simulink model "NDS_SKF"  (R2022b)
settings: Solver=ode4  StartTime=0.0  StopTime=10  RelTol=1e-3
values from neighbouring files (symbols this model uses):
  A = [(-2 * DCR * wn) -(wn^2); 1 0]    [NDS_SKFmat.m]
  B = [wn^2; 0]    [NDS_SKFmat.m]
  F_k1 = sys_d.A    [NDS_SKFmat.m]
  G_k1 = sys_d.B    [NDS_SKFmat.m]
  H_k1 = sys_d.C    [NDS_SKFmat.m]
  L_k1 = G_k1    [NDS_SKFmat.m]
  M_k1 = 1    [NDS_SKFmat.m]
  Pk0 = eye(size(xhat0, 1))    [NDS_SKFmat.m]
  Q = 0.1    [NDS_SKFmat.m]
  R = 0.1    [NDS_SKFmat.m]
  x0 = 0.5    [NDS_SKFmat.m]
  xdot0 = -0.01    [NDS_SKFmat.m]
  xhat0 = [0; 0]    [NDS_SKFmat.m]
settings Model: Creator=nathaliadesouza  LastModifiedBy=nathaliadesouza

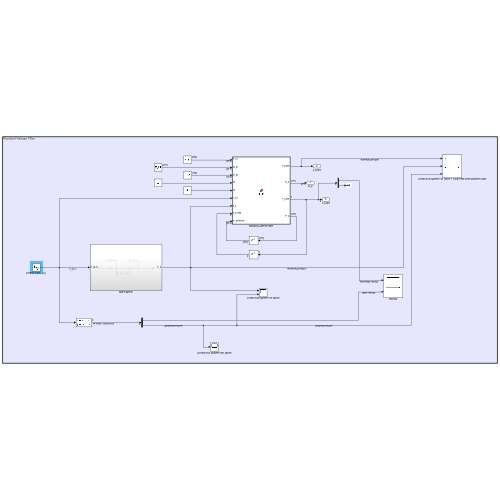
[thumbnail: Simulink's stored preview of the top-level diagram]
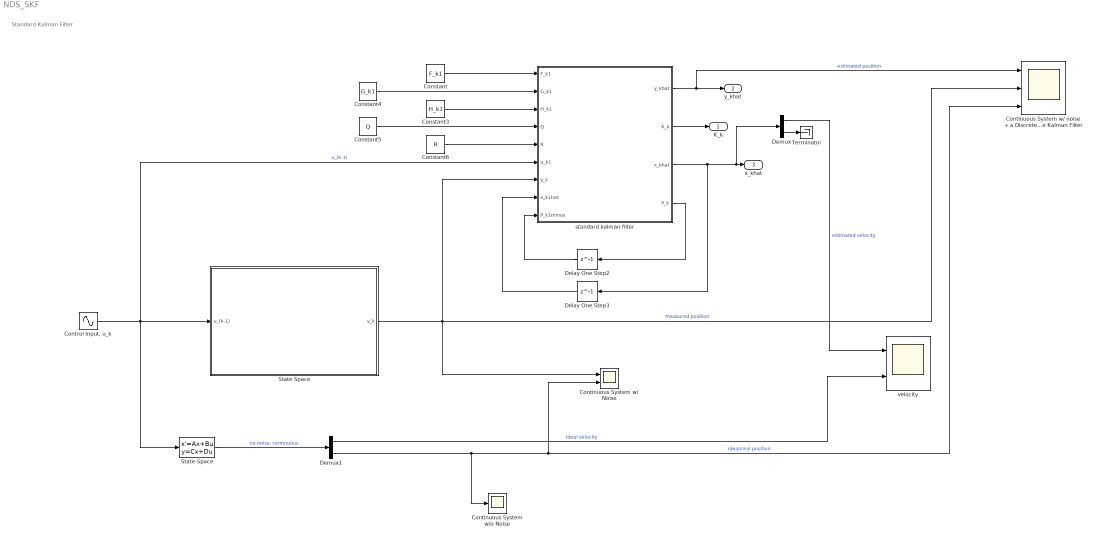
== system NDS_SKF ==
  note: Standard Kalman Filter
  Constant : Constant  Value=F_k1  VectorParams1D=off
  Constant3 : Constant  Value=H_k1  VectorParams1D=off
  Constant4 : Constant  Value=G_k1  VectorParams1D=off
  Constant5 : Constant  Value=Q
  Constant6 : Constant  Value=R
  Continuous System w/ Noise : Scope  NumInputPorts=2
  Continuous System w/ noise + a Discrete Time Kalman Filter : Scope  NumInputPorts=3
  Continuous System w/o Noise : Scope
  "Control Input, u_k " : Sin  SampleTime=0.1
  Delay One Step2 : Delay  DelayLength=1  InitialCondition=Pk0  SampleTime=0.1
  Delay One Step3 : Delay  DelayLength=1  InitialCondition=xhat0  SampleTime=0.1
  Demux : Demux  Outputs=2
  Demux1 : Demux  Outputs=2
  State Space : Subsystem
  State-Space : StateSpace  A=A  B=B  C=eye(2)  D=[0; 0]  InitialCondition=[x0 xdot0]
  Terminator : Terminator
  standard kalman filter : MATLAB Function  TreatAsAtomicUnit=on
  velocity : Scope  NumInputPorts=2
  K_k : Outport
  y_khat : Outport  Port=2
  x_khat : Outport  Port=3
  wires:
  "Control Input, u_k "/1 -> standard kalman filter/6(u_k1), State Space/1(u_(k-1)), State-Space/1  "u_(k-1)"
  Constant4/1 -> standard kalman filter/2(G_k1)
  Constant5/1 -> standard kalman filter/4(Q)
  Constant/1 -> standard kalman filter/1(F_k1)
  Constant6/1 -> standard kalman filter/5(R)
  Constant3/1 -> standard kalman filter/3(H_k1)
  standard kalman filter/3(x_khat) -> Delay One Step3/1, Demux/1, x_khat/1
  Delay One Step2/1 -> standard kalman filter/9(P_k1minus)
  Delay One Step3/1 -> standard kalman filter/8(x_k1hat)
  standard kalman filter/4(P_k) -> Delay One Step2/1
  standard kalman filter/1(y_khat) -> Continuous System w/ noise + a Discrete Time Kalman Filter/1, y_khat/1  "estimated position"
  standard kalman filter/2(K_k) -> K_k/1
  State-Space/1 -> Demux1/1  "no noise, continuous"
  Demux1/2 -> Continuous System w/o Noise/1, Continuous System w/ Noise/2, Continuous System w/ noise + a Discrete Time Kalman Filter/3  "ideal/real position"
  Demux1/1 -> velocity/2  "ideal velocity"
  Demux/1 -> velocity/1  "estimated velocity"
  Demux/2 -> Terminator/1
  State Space/1(y_k) -> standard kalman filter/7(y_k), Continuous System w/ Noise/1, Continuous System w/ noise + a Discrete Time Kalman Filter/2  "measured position"

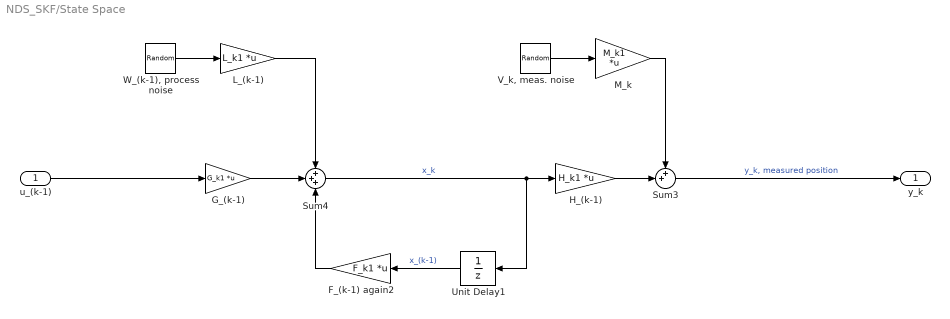
== system NDS_SKF/State Space ==
  u_(k-1) : Inport
  F_(k-1) again2 : Gain  Gain=F_k1  Multiplication=Matrix(K*u)
  G_(k-1) : Gain  Gain=G_k1  Multiplication=Matrix(K*u)
  H_(k-1) : Gain  Gain=H_k1  Multiplication=Matrix(K*u)
  L_(k-1) : Gain  Gain=L_k1  Multiplication=Matrix(K*u)  SampleTime=0.1
  M_k : Gain  Gain=M_k1  Multiplication=Matrix(K*u)  SampleTime=0.1
  Sum3 : Sum  Inputs=++|
  Sum4 : Sum  Inputs=+++
  Unit Delay1 : UnitDelay  InitialCondition=[0.5; -0.01]  SampleTime=0.1  HasFrameUpgradeWarning=on
  "V_k, meas. noise" : RandomNumber  Variance=0.01  SampleTime=0.1
  "W_(k-1), process noise" : RandomNumber  Variance=0.01  SampleTime=0.1
  y_k : Outport
  wires:
  u_(k-1)/1 -> G_(k-1)/1
  L_(k-1)/1 -> Sum4/1
  Unit Delay1/1 -> F_(k-1) again2/1  "x_(k-1)"
  "V_k, meas. noise"/1 -> M_k/1
  Sum4/1 -> Unit Delay1/1, H_(k-1)/1  "x_k"
  Sum3/1 -> y_k/1  "y_k, measured position"
  H_(k-1)/1 -> Sum3/2
  F_(k-1) again2/1 -> Sum4/3
  M_k/1 -> Sum3/1
  G_(k-1)/1 -> Sum4/2
  "W_(k-1), process noise"/1 -> L_(k-1)/1

== matlab function NDS_SKF/standard kalman filter ==
  data: y_khat output; K_k output; x_khat output; F_k1 input; G_k1 input; H_k1 input; Q input; R input; u_k1 input; y_k input; x_k1hat input; P_k1minus input; P_k output
function [y_khat, K_k, x_khat, P_k] = SKF(F_k1, G_k1, H_k1, Q, R,  u_k1, y_k, x_k1hat, P_k1minus)


% prediction step
x_kminushat = (F_k1 * x_k1hat) + (G_k1 * u_k1); % a priori state estimate
P_kminus = (F_k1 * P_k1minus * transpose(F_k1)) + (G_k1 * Q * G_k1'); % a priori covariance

% correction step
W = (H_k1 * P_kminus * transpose(H_k1)) + (H_k1 * R * transpose(H_k1));
K_k = P_kminus * transpose(H_k1) * (W^-1); % kalman gain
y_kminushat = H_k1 * x_kminushat; % predicted measurement given the a priori estimate
x_khat = x_kminushat + (K_k .* (y_k - y_kminushat)); % linear correction/update equation
P_k = P_kminus - (K_k * H_k1 * P_kminus) - (P_kminus * transpose(H_k1) * transpose(K_k)) + (K_k * W * transpose(K_k)); % a posteriori covariance
 
% estimation
y_khat = H_k1 * x_khat; % output estimaton
